simulink model "Logical_Architecture"  (R2025b)
settings: Solver=VariableStepAuto  StartTime=0.0  StopTime=10.0  RelTol=1e-3
settings Model: Creator=shrig  LastModifiedBy=shrig

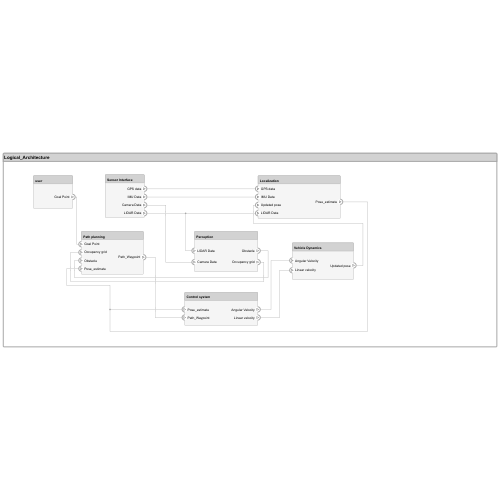
[thumbnail: Simulink's stored preview of the top-level diagram]
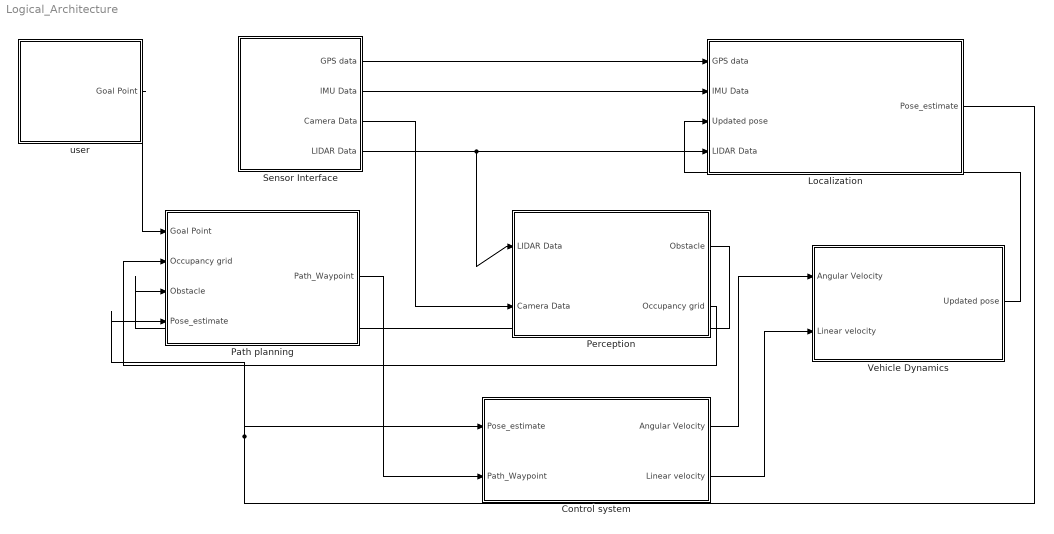
== system Logical_Architecture ==
  "Control system " : Subsystem
      settings: PortSchema="{\"entries\":[{\"content\":{\"headerSize\":26,\"margin\":15,\"minimumSpacing\":25,\"sides\":[{\"content\":{\"connectorIds\":[\"In1\",\"In2\"]},\"type\":\"ConnectorPlacement.EquallySpacedRectSide\",\"uuid\":\"79d1b898-d68d-468f-bdff-4613dd68d253\"},{\"content\":{\"connectorIds\":[\"Out1\",\"Out2\"],\"side\":\"RIGHT\"},\"type\":\"ConnectorPlacement.EquallySpacedRectSide\",\"uuid\":\"797d9a15-40ef-4c5f-a20d-7960b9ce3372\"},{\"content\":{\"side\":\"TOP\"},\"type\":\"ConnectorPlacement.EquallySpacedRectSide\",\"uuid\":\"bbf65513-0dd9-4c4f-ada8-84a57afa52a5\"}]},\"type\":\"ConnectorPlacement.EquallySpacedConnector\",\"uuid\":\"3b4a3355-3e94-4d3c-b478-af080979d33d\"}],\"packageUris\":[\"http://schema.mathworks.com/mf0/Connector/R2020b\"],\"version\":\"1.0\"}"
  "Localization " : Subsystem
      settings: PortSchema="{\"entries\":[{\"content\":{\"headerSize\":26,\"margin\":15,\"minimumSpacing\":25,\"sides\":[{\"content\":{\"connectorIds\":[\"In1\",\"In2\",\"In3\",\"In4\"]},\"type\":\"ConnectorPlacement.EquallySpacedRectSide\",\"uuid\":\"79d1b898-d68d-468f-bdff-4613dd68d253\"},{\"content\":{\"connectorIds\":[\"Out1\"],\"side\":\"RIGHT\"},\"type\":\"ConnectorPlacement.EquallySpacedRectSide\",\"uuid\":\"797d9a15-40ef-4c5f-a20d-7960b9ce3372\"},{\"content\":{\"side\":\"TOP\"},\"type\":\"ConnectorPlacement.EquallySpacedRectSide\",\"uuid\":\"bbf65513-0dd9-4c4f-ada8-84a57afa52a5\"}]},\"type\":\"ConnectorPlacement.EquallySpacedConnector\",\"uuid\":\"3b4a3355-3e94-4d3c-b478-af080979d33d\"}],\"packageUris\":[\"http://schema.mathworks.com/mf0/Connector/R2020b\"],\"version\":\"1.0\"}"
  Path planning : Subsystem
      settings: PortSchema="{\"entries\":[{\"content\":{\"headerSize\":26,\"margin\":15,\"minimumSpacing\":25,\"sides\":[{\"content\":{\"connectorIds\":[\"In1\",\"In2\",\"In3\",\"In4\"]},\"type\":\"ConnectorPlacement.EquallySpacedRectSide\",\"uuid\":\"79d1b898-d68d-468f-bdff-4613dd68d253\"},{\"content\":{\"connectorIds\":[\"Out1\"],\"side\":\"RIGHT\"},\"type\":\"ConnectorPlacement.EquallySpacedRectSide\",\"uuid\":\"797d9a15-40ef-4c5f-a20d-7960b9ce3372\"},{\"content\":{\"side\":\"TOP\"},\"type\":\"ConnectorPlacement.EquallySpacedRectSide\",\"uuid\":\"bbf65513-0dd9-4c4f-ada8-84a57afa52a5\"}]},\"type\":\"ConnectorPlacement.EquallySpacedConnector\",\"uuid\":\"3b4a3355-3e94-4d3c-b478-af080979d33d\"}],\"packageUris\":[\"http://schema.mathworks.com/mf0/Connector/R2020b\"],\"version\":\"1.0\"}"
  "Perception " : Subsystem
      settings: PortSchema="{\"entries\":[{\"content\":{\"headerSize\":26,\"margin\":15,\"minimumSpacing\":25,\"sides\":[{\"content\":{\"connectorIds\":[\"In1\",\"In2\"]},\"type\":\"ConnectorPlacement.EquallySpacedRectSide\",\"uuid\":\"79d1b898-d68d-468f-bdff-4613dd68d253\"},{\"content\":{\"connectorIds\":[\"Out1\",\"Out2\"],\"side\":\"RIGHT\"},\"type\":\"ConnectorPlacement.EquallySpacedRectSide\",\"uuid\":\"797d9a15-40ef-4c5f-a20d-7960b9ce3372\"},{\"content\":{\"side\":\"TOP\"},\"type\":\"ConnectorPlacement.EquallySpacedRectSide\",\"uuid\":\"bbf65513-0dd9-4c4f-ada8-84a57afa52a5\"}]},\"type\":\"ConnectorPlacement.EquallySpacedConnector\",\"uuid\":\"3b4a3355-3e94-4d3c-b478-af080979d33d\"}],\"packageUris\":[\"http://schema.mathworks.com/mf0/Connector/R2020b\"],\"version\":\"1.0\"}"
  Sensor Interface : Subsystem
      settings: PortSchema="{\"entries\":[{\"content\":{\"headerSize\":26,\"margin\":15,\"minimumSpacing\":25,\"sides\":[{\"content\":{},\"type\":\"ConnectorPlacement.EquallySpacedRectSide\",\"uuid\":\"79d1b898-d68d-468f-bdff-4613dd68d253\"},{\"content\":{\"connectorIds\":[\"Out1\",\"Out2\",\"Out3\",\"Out4\"],\"side\":\"RIGHT\"},\"type\":\"ConnectorPlacement.EquallySpacedRectSide\",\"uuid\":\"797d9a15-40ef-4c5f-a20d-7960b9ce3372\"},{\"content\":{\"side\":\"TOP\"},\"type\":\"ConnectorPlacement.EquallySpacedRectSide\",\"uuid\":\"bbf65513-0dd9-4c4f-ada8-84a57afa52a5\"}]},\"type\":\"ConnectorPlacement.EquallySpacedConnector\",\"uuid\":\"3b4a3355-3e94-4d3c-b478-af080979d33d\"}],\"packageUris\":[\"http://schema.mathworks.com/mf0/Connector/R2020b\"],\"version\":\"1.0\"}"
  Vehicle Dynamics : Subsystem
      settings: PortSchema="{\"entries\":[{\"content\":{\"headerSize\":26,\"margin\":15,\"minimumSpacing\":25,\"sides\":[{\"content\":{\"connectorIds\":[\"In1\",\"In2\"]},\"type\":\"ConnectorPlacement.EquallySpacedRectSide\",\"uuid\":\"79d1b898-d68d-468f-bdff-4613dd68d253\"},{\"content\":{\"connectorIds\":[\"Out1\"],\"side\":\"RIGHT\"},\"type\":\"ConnectorPlacement.EquallySpacedRectSide\",\"uuid\":\"797d9a15-40ef-4c5f-a20d-7960b9ce3372\"},{\"content\":{\"side\":\"TOP\"},\"type\":\"ConnectorPlacement.EquallySpacedRectSide\",\"uuid\":\"bbf65513-0dd9-4c4f-ada8-84a57afa52a5\"}]},\"type\":\"ConnectorPlacement.EquallySpacedConnector\",\"uuid\":\"3b4a3355-3e94-4d3c-b478-af080979d33d\"}],\"packageUris\":[\"http://schema.mathworks.com/mf0/Connector/R2020b\"],\"version\":\"1.0\"}"
  user : Subsystem
      settings: PortSchema="{\"entries\":[{\"content\":{\"headerSize\":26,\"margin\":15,\"minimumSpacing\":25,\"sides\":[{\"content\":{},\"type\":\"ConnectorPlacement.EquallySpacedRectSide\",\"uuid\":\"4819f95f-e283-4e7e-a97a-9ea20b5e0d92\"},{\"content\":{\"connectorIds\":[\"Out1\"],\"side\":\"RIGHT\"},\"type\":\"ConnectorPlacement.EquallySpacedRectSide\",\"uuid\":\"0e781af4-b96e-4a71-a1b8-f3bf53e8e4ad\"},{\"content\":{\"side\":\"TOP\"},\"type\":\"ConnectorPlacement.EquallySpacedRectSide\",\"uuid\":\"7018724f-dbfe-4407-9528-ea5e815360fe\"}]},\"type\":\"ConnectorPlacement.EquallySpacedConnector\",\"uuid\":\"54d63656-1d72-4fa5-b8ad-a175bdb4bffc\"}],\"packageUris\":[\"http://schema.mathworks.com/mf0/Connector/R2020b\"],\"version\":\"1.0\"}"
  wires:
  Sensor Interface/2(IMU Data) -> "Localization "/2(IMU Data)
  Sensor Interface/1(GPS data) -> "Localization "/1(GPS data)
  Sensor Interface/4(LIDAR Data) -> "Perception "/1(LIDAR Data), "Localization "/4(LIDAR Data)
  Sensor Interface/3(Camera Data) -> "Perception "/2(Camera Data)
  Path planning/1(Path_Waypoint) -> "Control system "/2(Path_Waypoint)
  "Localization "/1(Pose_estimate) -> Path planning/4(Pose_estimate), "Control system "/1(Pose_estimate)
  "Perception "/2(Occupancy grid) -> Path planning/2(Occupancy grid)
  "Control system "/2(Linear velocity) -> Vehicle Dynamics/2(Linear velocity)
  "Control system "/1(Angular Velocity) -> Vehicle Dynamics/1(Angular Velocity)
  Vehicle Dynamics/1(Updated pose) -> "Localization "/3(Updated pose)
  "Perception "/1(Obstacle) -> Path planning/3(Obstacle)
  user/1(Goal Point) -> Path planning/1(Goal Point)

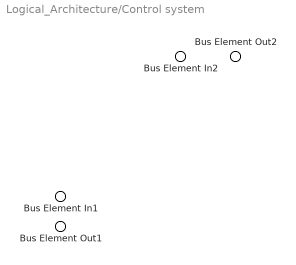
== system Logical_Architecture/Control system  ==
  Bus Element In2 : Inport  PortName=Pose_estimate
  Bus Element In1 : Inport  Port=2  PortName=Path_Waypoint
  Bus Element Out2 : Outport  PortName=Angular Velocity
  Bus Element Out1 : Outport  Port=2  PortName=Linear velocity

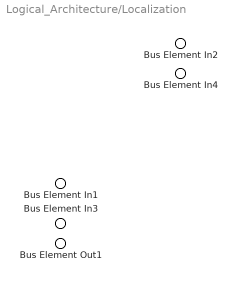
== system Logical_Architecture/Localization  ==
  Bus Element In2 : Inport  PortName=GPS data
  Bus Element In1 : Inport  Port=2  PortName=IMU Data
  Bus Element In4 : Inport  Port=3  PortName=Updated pose
  Bus Element In3 : Inport  Port=4  PortName=LIDAR Data
  Bus Element Out1 : Outport  PortName=Pose_estimate

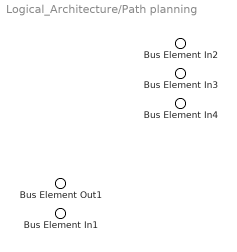
== system Logical_Architecture/Path planning ==
  Bus Element In3 : Inport  PortName=Goal Point
  Bus Element In2 : Inport  Port=2  PortName=Occupancy grid
  Bus Element In4 : Inport  Port=3  PortName=Obstacle
  Bus Element In1 : Inport  Port=4  PortName=Pose_estimate
  Bus Element Out1 : Outport  PortName=Path_Waypoint

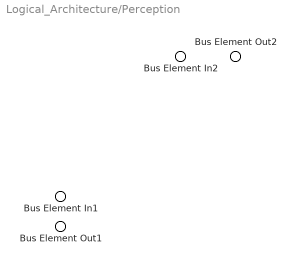
== system Logical_Architecture/Perception  ==
  Bus Element In2 : Inport  PortName=LIDAR Data
  Bus Element In1 : Inport  Port=2  PortName=Camera Data
  Bus Element Out2 : Outport  PortName=Obstacle
  Bus Element Out1 : Outport  Port=2  PortName=Occupancy grid

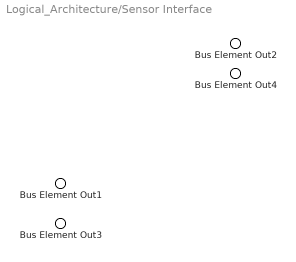
== system Logical_Architecture/Sensor Interface ==
  Bus Element Out2 : Outport  PortName=GPS data
  Bus Element Out1 : Outport  Port=2  PortName=IMU Data
  Bus Element Out4 : Outport  Port=3  PortName=Camera Data
  Bus Element Out3 : Outport  Port=4  PortName=LIDAR Data

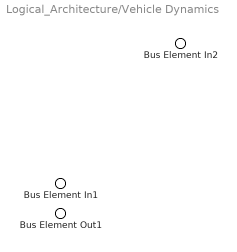
== system Logical_Architecture/Vehicle Dynamics ==
  Bus Element In2 : Inport  PortName=Angular Velocity
  Bus Element In1 : Inport  Port=2  PortName=Linear velocity
  Bus Element Out1 : Outport  PortName=Updated pose

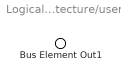
== system Logical_Architecture/user ==
  Bus Element Out1 : Outport  PortName=Goal Point
